simulink subsystem "s0315_alpha_theta_controller_PP_PID"  (R2019b)
settings: Solver=VariableStepAuto  StartTime=0.0  StopTime=10.0  RelTol=1e-3
model mask{p1=0, p2=0, p3=0, wc=0, cz_ratio=0, pc_ratio=0}
  mask prompts: p1 "Position 1st pole"; p2 "Position 2nd pole"; p3 "Position 3rd pole"; wc "PID cutting frequency"; cz_ratio "PID cutting/zeros ratio"; pc_ratio "PID pole/cutting ratio"
undefined symbols (not defined in the file): DiscIntNeverNeededParam, dt_control, PARAMS
libraries: simulink x2
settings Model: Creator=francescoceresetti  LastModifiedBy=francescoceresetti

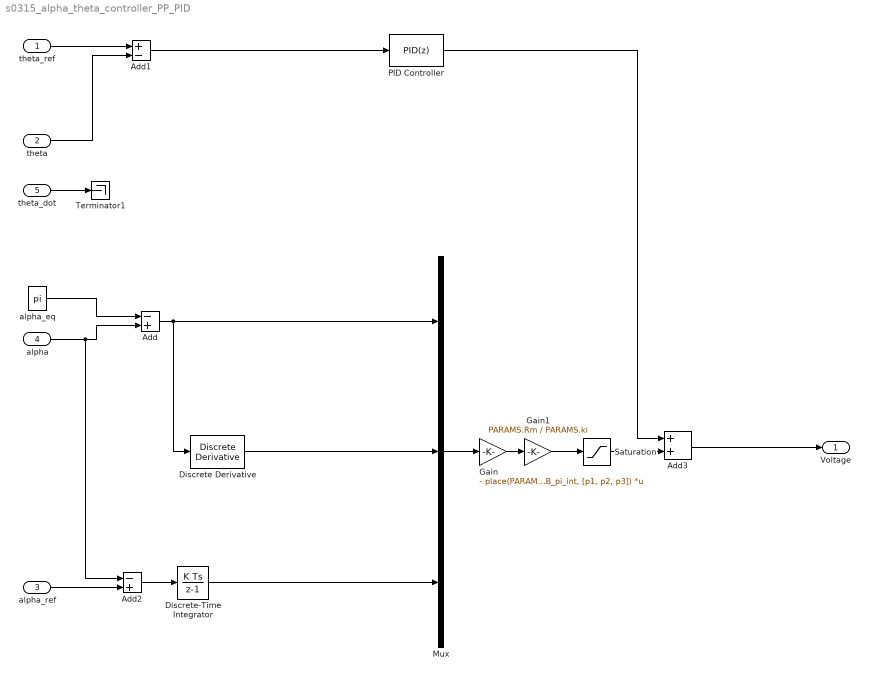
== system s0315_alpha_theta_controller_PP_PID ==
  theta_ref : Inport
  theta : Inport  Port=2
  alpha_ref : Inport  Port=3
  alpha : Inport  Port=4
  theta_dot : Inport  Port=5
  Add : Sum  Inputs=-+
  Add1 : Sum  Inputs=+-
  Add2 : Sum  Inputs=-+
  Add3 : Sum
  Discrete Derivative : simulink/Discrete/Discrete Derivative  gainval=1.0  ICPrevScaledInput=pi  OutMin=[]  OutMax=[]  OutDataType=fixdt(1, 16)  OutScaling=2^-10  DoSatur=off
  Discrete-Time Integrator : DiscreteIntegrator  SampleTime=-1  ICPrevOutput=DiscIntNeverNeededParam  ICPrevScaledInput=DiscIntNeverNeededParam
  Gain : Gain  Gain=- place(PARAMS.A_pi_int, PARAMS.B_pi_int, [p1, p2, p3])  Multiplication=Matrix(K*u)
  Gain1 : Gain  Gain=PARAMS.Rm / PARAMS.ki
  Mux : Mux  Inputs=3
  PID Controller : simulink/Continuous/PID Controller  Controller=PID  Form=Parallel  TimeDomain=Discrete-time  SampleTime=dt_control  IntegratorMethod=Forward Euler  FilterMethod=Forward Euler  ControllerParametersSource=internal  P=wc^2 * (2 * cz_ratio * pc_ratio - 1) / (cz_ratio^2 * pc_ratio * PARAMS.mu_V_theta_dot)  I=wc^3 / PARAMS.mu_V_theta_dot / cz_ratio^2  D="wc * (cz_ratio^2 * pc_ratio^2 - 2 * cz_ratio * pc_ratio + 1)  / (cz_ratio^2 * pc_ratio^2 * PARAMS.mu_V_theta_dot)"  UseFilter=on  N=pc_ratio * wc  TunerSelectOption=Transfer Function Based (PID Tuner App)  InitialConditionSource=internal  InitialConditionForIntegrator=0  InitialConditionForFilter=0  DifferentiatorICPrevScaledInput=0  ExternalReset=none  TrackingMode=off  Kt=1  LimitOutput=on  UpperSaturationLimit=PARAMS.V_sat  LowerSaturationLimit=-PARAMS.V_sat  LinearizeAsGain=on  AntiWindupMode=none  Kb=1  POutMin=[]  POutMax=[]  IOutMin=[]  IOutMax=[]  DOutMin=[]  DOutMax=[]  NOutMin=[]  NOutMax=[]  SumOutMin=[]  SumOutMax=[]  SaturationOutMin=[]  SaturationOutMax=[]  PParamMin=[]  PParamMax=[]  IParamMin=[]  IParamMax=[]  DParamMin=[]  DParamMax=[]  NParamMin=[]  NParamMax=[]  KbParamMin=[]  KbParamMax=[]  KtParamMin=[]  KtParamMax=[]  KbOutMin=[]  KbOutMax=[]  KtOutMin=[]  KtOutMax=[]  IntegratorOutMin=[]  IntegratorOutMax=[]  FilterOutMin=[]  FilterOutMax=[]  SumI1OutMin=[]  SumI1OutMax=[]  SumI2OutMin=[]  SumI2OutMax=[]  SumI3OutMin=[]  SumI3OutMax=[]  SumI4OutMin=[]  SumI4OutMax=[]  SumDOutMin=[]  SumDOutMax=[]  DifferentiatorOutMin=[]  DifferentiatorOutMax=[]  FilterDiffOutCoefMin=[]  FilterDiffOutCoefMax=[]  ReciprocalOutMin=[]  ReciprocalOutMax=[]  SumDenOutMin=[]  SumDenOutMax=[]  SumNumOutMin=[]  SumNumOutMax=[]  DivideOutMin=[]  DivideOutMax=[]  IntegratorContinuousStateAttributes=''  IntegratorStateMustResolveToSignalObject=off  IntegratorRTWStateStorageClass=Auto  FilterContinuousStateAttributes=''  FilterStateMustResolveToSignalObject=off  FilterRTWStateStorageClass=Auto  ParallelPVariant=InternalParameters  IdealPVariant=Disabled  IVariant=InternalParameters  DVariant=InternalParameters  IntegratorVariant=Discrete  SatVariant=Enabled  AWVariant=Passthrough  PCopyVariant=Disabled  TRVariant=Disabled  FdbkBlocksVariant=Forward  IdealPFdbkVariant=Disabled  SatFdbkVariant=Disabled  DerivativeFilterVariant=ForwardEulerFilter  NVariant=InternalParameters  NCopyVariant=Disabled  FilterICVariant=InternalICsFilter  IntegratorICVariant=InternalICs  ExternalResetVariant=Disabled  TRSumVariant=Passthrough  SumFdbkVariant=Disabled  SumVariant=Sum_PID
  Saturation : Saturate  UpperLimit=PARAMS.V_sat*0.7  LowerLimit=-PARAMS.V_sat*0.7
  Terminator1 : Terminator
  "alpha_eq " : Constant  Value=pi
  Voltage : Outport
  wires:
  theta_ref/1 -> Add1/1
  theta/1 -> Add1/2
  theta_dot/1 -> Terminator1/1
  alpha_ref/1 -> Add2/2
  Discrete-Time Integrator/1 -> Mux/3
  alpha/1 -> Add2/1, Add/2
  "alpha_eq "/1 -> Add/1
  Add/1 -> Mux/1, Discrete Derivative/1
  Gain/1 -> Gain1/1
  Add2/1 -> Discrete-Time Integrator/1
  Discrete Derivative/1 -> Mux/2
  Mux/1 -> Gain/1
  Add1/1 -> PID Controller/1
  Add3/1 -> Voltage/1
  PID Controller/1 -> Add3/1
  Gain1/1 -> Saturation/1
  Saturation/1 -> Add3/2
